simulink model "radar_sim"  (R2022a)
settings: Solver=VariableStepAuto  StartTime=0.0  StopTime=10.0  RelTol=1e-3
undefined symbols (not defined in the file or in its folder): phased, physconst
libraries: phasedtxrxlib x3, phasedwavlib x1, phasedenvlib x1
settings Model: Creator=Dayalan  LastModifiedBy=Dayalan

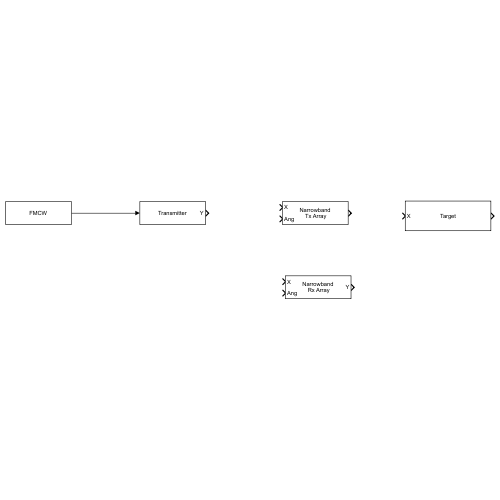
[thumbnail: Simulink's stored preview of the top-level diagram]
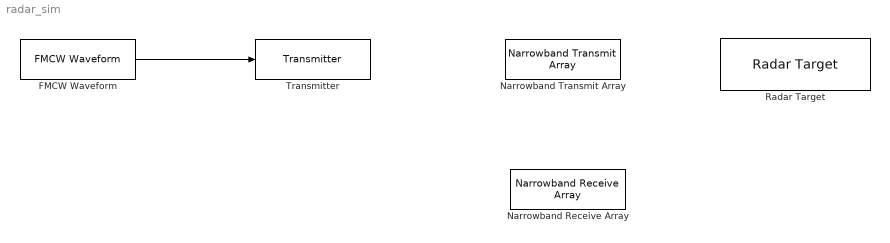
== system radar_sim ==
  FMCW Waveform : phasedwavlib/FMCW Waveform  SampleRate=1e6  SweepTime=1e-4  SweepBandwidth=1e5  SweepDirection=Up  SweepInterval=Positive  OutputFormat=Sweeps  NumSamples=100  NumSweeps=1  SimulateUsing=Interpreted execution
      settings: SourceProductBaseCode=AR
  Narrowband Receive Array : phasedtxrxlib/Narrowband Receive Array  PropagationSpeed=physconst( 'LightSpeed' )  OperatingFrequency=3e8  Wavefront=Plane  SensorGainMeasure=dB  Polarization=None  WeightsInputPort=off  SimulateUsing=Interpreted execution  Sensor=phased.ULA('Element',phased.IsotropicAntennaElement)
      settings: SourceProductBaseCode=AR
  Narrowband Transmit Array : phasedtxrxlib/Narrowband Transmit Array  PropagationSpeed=physconst( 'LightSpeed' )  OperatingFrequency=24e9  CombineRadiatedSignals=on  SensorGainMeasure=dB  Polarization=None  WeightsInputPort=off  SimulateUsing=Interpreted execution  Sensor=phased.ULA('Element',phased.IsotropicAntennaElement)
      settings: SourceProductBaseCode=AR
  Radar Target : phasedenvlib/Radar Target  EnablePolarization=off  Mode=Monostatic  MeanRCSSource=Property  ScatteringMatrixSource=Property  MeanRCS=1  ScatteringMatrix=eye( 2 )  Model=Nonfluctuating  PropagationSpeed=physconst( 'LightSpeed' )  OperatingFrequency=3e8  SeedSource=Auto  Seed=0  SimulateUsing=Interpreted execution
      settings: SourceProductBaseCode=AR
  Transmitter : phasedtxrxlib/Transmitter  PeakPower=5000  Gain=20  LossFactor=0  InUseOutputPort=off  CoherentOnTransmit=on  PhaseNoiseOutputPort=off  SeedSource=Auto  Seed=0  SimulateUsing=Interpreted execution
      settings: SourceProductBaseCode=AR
  wires:
  FMCW Waveform/1 -> Transmitter/1
